simulink model "Seri_HEV_Model"  (R2025b)
settings: Solver=ode23t  StartTime=0.0  StopTime=2474  RelTol=1e-3
values from neighbouring files (symbols this model uses):
  Bat_Capacity_Ah = 30    [Seri_ve_Paralel_Hibrit_Proje.m]
  SOC_initial = 0.60    (= 0.6)    [Seri_ve_Paralel_Hibrit_Proje.m]
libraries: fl_lib x6, sdl_lib x4, nesl_utility x3, autolibshared x2, autolibmappedmotor x2, autolibdatasheetbattery x1, autolibsharedmappedengines x1
(part 4 of 4)

== stateflow chart Seri_HEV_Model/Kontrolcü ==
  state EV_Modu
    du:
    Trq_ICE = 0;
    Trq_EM = Accel * 300;
  state Hibrit_Modu
    du: Trq_ICE = 80;
    Trq_EM = Accel * 300;
  state Frenleme
    du:
    Trq_ICE = 0;
    Trq_EM = -Decel * 300;
  (default) -> EV_Modu
  EV_Modu -> Frenleme [order 3] : [Decel > 0]
  Frenleme -> EV_Modu [order 1] : [Decel == 0 && SOC>0.59]
  EV_Modu -> Hibrit_Modu [order 1] : [ SOC <= 0.59]
  EV_Modu -> Frenleme [order 2] : [Decel > 0]
  Hibrit_Modu -> EV_Modu [order 1] : [SOC >= 0.65]
  Hibrit_Modu -> Frenleme [order 2] : [Decel > 0]
  Frenleme -> Hibrit_Modu [order 2] : [Decel == 0 && SOC <= 0.59]
  data: Decel input; Accel input; SOC input; V input; Trq_EM output; Trq_ICE output
